simulink model "ctrl_T"  (R2015a)
settings: Solver=ode3  StartTime=0.0  StopTime=inf  FixedStep=0.01  RelTol=1e-3
values from neighbouring files (symbols this model uses):
  C = [C1;C2;C3;C4;C5;C6]    [initfile.m]    (also in thrustallocationQuadraticFixed.m)
  D = 3.0/100    (= 0.03)    [initfile.m]    (also in thrustallocationQuadraticFixed.m = 0.0411111111111)
  eps_c = 5    [initfile.m]
  epsilon = 0.5    [initfile.m]    (also in thrustallocationPseudo.m = u(10); thrustallocationQuadraticFixed.m = u(10))
  hd = c2d(H1,0.01,'foh')    [initfile.m]
  hd2 = c2d(H2,0.01,'zoh')    [initfile.m]
  I_s = 25000 /747225    (= 0.0334571246947)    [initfile.m]
  k_cc = 1    [initfile.m]
  K_omega = 0.3    [initfile.m]
  Kp = 3.3    [initfile.m]
  Max_Acceleration = 5    [initfile.m]
  Max_rotation = 12*sqrt(lambda)    [initfile.m]
  Max_thrust = 1.5    [initfile.m]
  n_c = 5    [initfile.m]
  n_max = 152    [initfile.m]
  p_cc = 0.5    [initfile.m]
  Q_f0 = 0.3    [initfile.m]
  r_cc = 4    [initfile.m]
  Rho = Rho_m    (= 1000)    [initfile.m]
undefined symbols (not defined in the file or in its folder): Kq, Kqr, Kt, Ktr, P_max, Q_max, shaft_to_pwm_coeff, thrust_to_pwm_coeff, Thruster, Thruster_control, Thruster_lock
libraries: simulink x6, marine_gnc x4, simulink_extras x3
(part 3 of 4)

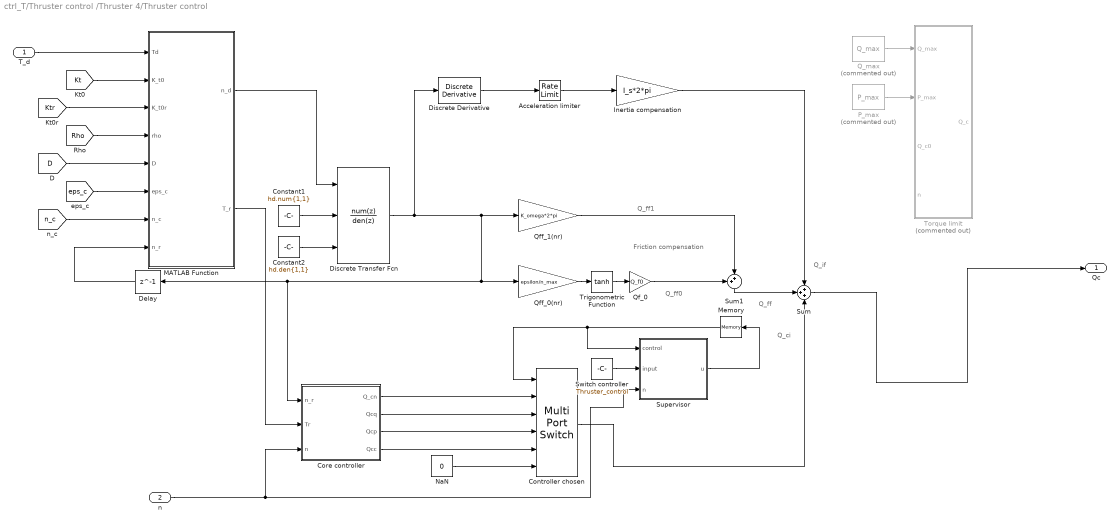
== system ctrl_T/Thruster control /Thruster 4/Thruster control ==
  note: Q_ci
  note: Q_if
  note: Q_ff
  note: Q_ff0
  note: Q_ff1
  note: Friction compensation
  "T_d " : Inport
  n : Inport  Port=2
  Acceleration limiter : RateLimiter  RisingSlewLimit=Max_Acceleration  FallingSlewLimit=-Max_Acceleration  SampleTimeMode=inherited
  Constant1 : Constant  Value=hd.num{1,1}  VectorParams1D=off
  Constant2 : Constant  Value=hd.den{1,1}  VectorParams1D=off
  Controller chosen : MultiPortSwitch  Inputs=5
  Core controller : Subsystem
  Delay : Delay  DelayLength=1  InitialCondition=0
  Discrete Transfer Fcn : DiscreteTransferFcn  NumeratorSource=Input port  Numerator=[8.76e-05 0.0003481 8.648e-05]  DenominatorSource=Input port  Denominator=[1 -1.974 0.9746]  SampleTime=0.01  a0EqualsOne=on
      settings: InputPortMap=u0,p1,p3
  Discrete Derivative : simulink/Discrete/Discrete Derivative  gainval=1.0  ICPrevScaledInput=0.0  InputProcessing=Inherited  OutMin=[]  OutMax=[]  OutDataType=fixdt(1, 16)  OutScaling=2^-10  DoSatur=off
  Inertia compensation : Gain  Gain=I_s*2*pi
  MATLAB Function : MATLAB Function  TreatAsAtomicUnit=on
  Memory : Memory  X0=1
  NaN : Constant  Value=0
  P_max : Constant  Commented=on  Value=P_max
  Q_max : Constant  Commented=on  Value=Q_max
  Qf_0 : Gain  Gain=Q_f0
  Qff_0(nr) : Gain  Gain=epsilon/n_max
  Qff_1(nr) : Gain  Gain=K_omega*2*pi
  Sum : Sum  Inputs=+++
  Sum1 : Sum  Inputs=++|
  Supervisor : MATLAB Function  TreatAsAtomicUnit=on
  Switch controller : Constant  Value=Thruster_control
  Torque limit : MATLAB Function  Commented=on  TreatAsAtomicUnit=on
  Trigonometric Function : Trigonometry  Operator=tanh
  Qc : Outport
  wires:
  P_max/1 -> Torque limit/2(P_max)
  Q_max/1 -> Torque limit/1(Q_max)
  Sum/1 -> Qc/1
  MATLAB Function/2(T_r) -> Core controller/2("Tr ")
  Discrete Derivative/1 -> Acceleration limiter/1
  Qff_0(nr)/1 -> Trigonometric Function/1
  Trigonometric Function/1 -> Qf_0/1
  Sum1/1 -> Sum/2
  Core controller/1(Q_cn) -> Controller chosen/2
  Core controller/4(Qcc) -> Controller chosen/5
  NaN/1 -> Controller chosen/6
  Memory/1 -> Supervisor/1(control), Controller chosen/1
  Qff_1(nr)/1 -> Sum1/2
  Qf_0/1 -> Sum1/1
  Controller chosen/1 -> Sum/3
  Inertia compensation/1 -> Sum/1
  Core controller/3(Qcp) -> Controller chosen/4
  Core controller/2(Qcq) -> Controller chosen/3
  Switch controller/1 -> Supervisor/2(input)
  "T_d "/1 -> MATLAB Function/1(Td)
  [Kt] -> MATLAB Function/2(K_t0)
  [Rho] -> MATLAB Function/4(rho)
  [D] -> MATLAB Function/5(D)
  [eps_c] -> MATLAB Function/6(eps_c)
  [Ktr] -> MATLAB Function/3(K_t0r)
  [n_c] -> MATLAB Function/7(n_c)
  Constant1/1 -> Discrete Transfer Fcn/2
  Constant2/1 -> Discrete Transfer Fcn/3
  MATLAB Function/1(n_d) -> Discrete Transfer Fcn/1
  n/1 -> Supervisor/3(n), Core controller/3("n ")
  Discrete Transfer Fcn/1 -> Discrete Derivative/1, Core controller/1(n_r), Delay/1, Qff_0(nr)/1, Qff_1(nr)/1
  Acceleration limiter/1 -> Inertia compensation/1
  Supervisor/1(u) -> Memory/1
  Delay/1 -> MATLAB Function/8(n_r)

== system ctrl_T/Thruster control /Thruster 5/Propeller Hydrodynamics ==
  env : Inport
  n : Inport  Port=2
  Actual Force and Torque : MATLAB Function  TreatAsAtomicUnit=on
  Ta : Outport
  Qa : Outport  Port=2
  wires:
  n/1 -> Actual Force and Torque/1(n)
  [D] -> Actual Force and Torque/7(D)
  [Kq] -> Actual Force and Torque/2(Kq)
  Actual Force and Torque/2(Qa) -> Qa/1
  [Rho] -> Actual Force and Torque/6(Rho)
  env/1 -> Actual Force and Torque/9(env)
  [Kt] -> Actual Force and Torque/3(Kt)
  Actual Force and Torque/1(Ta) -> Ta/1
  [Ktr] -> Actual Force and Torque/4(Ktr)
  [Kqr] -> Actual Force and Torque/5(Kqr)
  [eps_c] -> Actual Force and Torque/8(eps_c)

== system ctrl_T/Thruster control /Thruster 5/Shaft dynamics ==
  Qm : Inport
  Qa : Inport  Port=2
  Finding rotation speed : Gain  Gain=1/(2*pi*I_s)
  Integrator : Integrator  ExternalReset=either
  K_omega : Gain  Gain=K_omega*2*pi
  Sum : Sum  Inputs=-+-
  reset : S-Function  Priority=1  FunctionName=NIVeriStandIO  Parameters=width dtype portnum stime stype btype  mask(NI VeriStand Inport){portnum=1, width=-1, stime=-1, dtype=auto, stype=auto, btype=1}
      mask prompts: portnum "Port number:"; width "Port dimensions (-1 for dynamically sized):"; stime "Sample time (-1 for inherited):"; dtype "Data type:"; stype "Signal type:"; btype "Block type:"
      mask help: Use this inport on any level of nested subsystems to allow NI VeriStand software to map signals to it.
      mask init:
      | NIVeriStandIO_init;
      settings: CopyFcn=NIVeriStand_MDL_functions('', 'IO_copy');  DeleteFcn=NIVeriStand_MDL_functions('', 'IO_delete');  MoveFcn=set_param(gcb, 'Mask', 'on');
      mask Callback portnum: NIVeriStand_MDL_functions('', 'IO_setportnum');
      mask TypeOptions dtype: auto | double | single | int8 | uint8 | int16 | uint16 | int32 | uint32 | boolean
      mask Callback dtype: NIVeriStand_MDL_functions('', 'IO_booleansignal');
      mask TypeOptions stype: auto | real | complex
      mask Display:
      | patch([-x x], [-y y], [.90980 .81960 .32156]);
      | plot([xrad -x x xrad], [yrad -y y yrad]);
      | fprintf('NI In%d', portnum);
  n : Outport
  wires:
  Qm/1 -> Sum/2
  Sum/1 -> Finding rotation speed/1
  Qa/1 -> Sum/1
  K_omega/1 -> Sum/3
  Finding rotation speed/1 -> Integrator/1
  Integrator/1 -> K_omega/1, n/1
  reset/1 -> Integrator/2

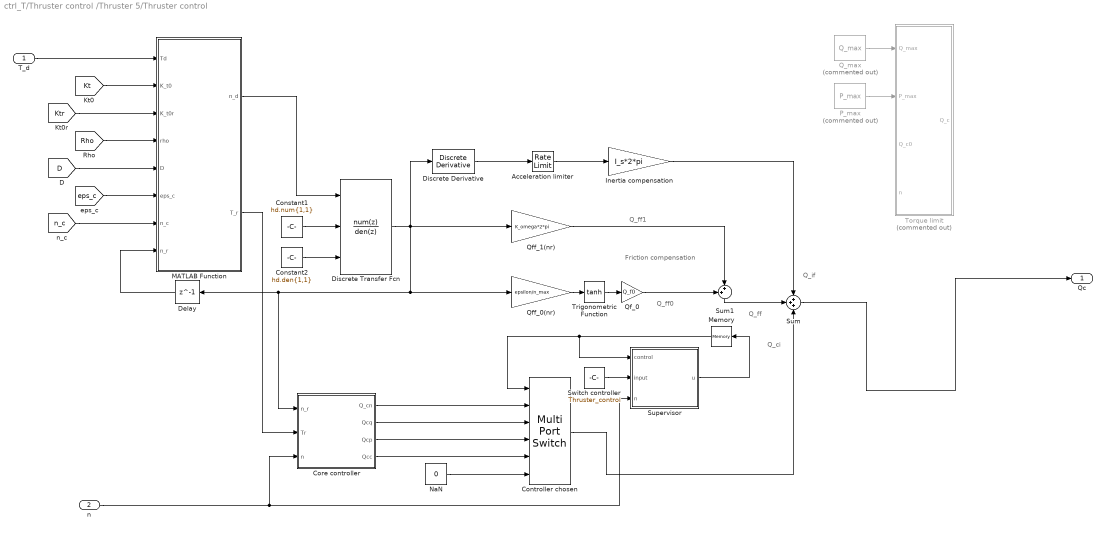
== system ctrl_T/Thruster control /Thruster 5/Thruster control ==
  note: Q_ci
  note: Q_if
  note: Q_ff
  note: Q_ff0
  note: Q_ff1
  note: Friction compensation
  "T_d " : Inport
  n : Inport  Port=2
  Acceleration limiter : RateLimiter  RisingSlewLimit=Max_Acceleration  FallingSlewLimit=-Max_Acceleration  SampleTimeMode=inherited
  Constant1 : Constant  Value=hd.num{1,1}  VectorParams1D=off
  Constant2 : Constant  Value=hd.den{1,1}  VectorParams1D=off
  Controller chosen : MultiPortSwitch  Inputs=5
  Core controller : Subsystem
  Delay : Delay  DelayLength=1  InitialCondition=0
  Discrete Transfer Fcn : DiscreteTransferFcn  NumeratorSource=Input port  Numerator=[8.76e-05 0.0003481 8.648e-05]  DenominatorSource=Input port  Denominator=[1 -1.974 0.9746]  SampleTime=0.01  a0EqualsOne=on
      settings: InputPortMap=u0,p1,p3
  Discrete Derivative : simulink/Discrete/Discrete Derivative  gainval=1.0  ICPrevScaledInput=0.0  InputProcessing=Inherited  OutMin=[]  OutMax=[]  OutDataType=fixdt(1, 16)  OutScaling=2^-10  DoSatur=off
  Inertia compensation : Gain  Gain=I_s*2*pi
  MATLAB Function : MATLAB Function  TreatAsAtomicUnit=on
  Memory : Memory  X0=1
  NaN : Constant  Value=0
  P_max : Constant  Commented=on  Value=P_max
  Q_max : Constant  Commented=on  Value=Q_max
  Qf_0 : Gain  Gain=Q_f0
  Qff_0(nr) : Gain  Gain=epsilon/n_max
  Qff_1(nr) : Gain  Gain=K_omega*2*pi
  Sum : Sum  Inputs=+++
  Sum1 : Sum  Inputs=++|
  Supervisor : MATLAB Function  TreatAsAtomicUnit=on
  Switch controller : Constant  Value=Thruster_control
  Torque limit : MATLAB Function  Commented=on  TreatAsAtomicUnit=on
  Trigonometric Function : Trigonometry  Operator=tanh
  Qc : Outport
  wires:
  P_max/1 -> Torque limit/2(P_max)
  Q_max/1 -> Torque limit/1(Q_max)
  Sum/1 -> Qc/1
  MATLAB Function/2(T_r) -> Core controller/2("Tr ")
  Discrete Derivative/1 -> Acceleration limiter/1
  Qff_0(nr)/1 -> Trigonometric Function/1
  Trigonometric Function/1 -> Qf_0/1
  Sum1/1 -> Sum/2
  Core controller/1(Q_cn) -> Controller chosen/2
  Core controller/4(Qcc) -> Controller chosen/5
  NaN/1 -> Controller chosen/6
  Memory/1 -> Supervisor/1(control), Controller chosen/1
  Qff_1(nr)/1 -> Sum1/2
  Qf_0/1 -> Sum1/1
  Controller chosen/1 -> Sum/3
  Inertia compensation/1 -> Sum/1
  Core controller/3(Qcp) -> Controller chosen/4
  Core controller/2(Qcq) -> Controller chosen/3
  Switch controller/1 -> Supervisor/2(input)
  "T_d "/1 -> MATLAB Function/1(Td)
  [Kt] -> MATLAB Function/2(K_t0)
  [Rho] -> MATLAB Function/4(rho)
  [D] -> MATLAB Function/5(D)
  [eps_c] -> MATLAB Function/6(eps_c)
  [Ktr] -> MATLAB Function/3(K_t0r)
  [n_c] -> MATLAB Function/7(n_c)
  Constant1/1 -> Discrete Transfer Fcn/2
  Constant2/1 -> Discrete Transfer Fcn/3
  MATLAB Function/1(n_d) -> Discrete Transfer Fcn/1
  Discrete Transfer Fcn/1 -> Discrete Derivative/1, Qff_0(nr)/1, Core controller/1(n_r), Delay/1, Qff_1(nr)/1
  Acceleration limiter/1 -> Inertia compensation/1
  Supervisor/1(u) -> Memory/1
  Delay/1 -> MATLAB Function/8(n_r)
  n/1 -> Core controller/3("n "), Supervisor/3(n)

== system ctrl_T/Thruster control /Thruster 6/Propeller Hydrodynamics ==
  env : Inport
  n : Inport  Port=2
  Actual Force and Torque : MATLAB Function  TreatAsAtomicUnit=on
  Ta : Outport
  Qa : Outport  Port=2
  wires:
  n/1 -> Actual Force and Torque/1(n)
  [D] -> Actual Force and Torque/7(D)
  [Kq] -> Actual Force and Torque/2(Kq)
  Actual Force and Torque/2(Qa) -> Qa/1
  [Rho] -> Actual Force and Torque/6(Rho)
  env/1 -> Actual Force and Torque/9(env)
  [Kt] -> Actual Force and Torque/3(Kt)
  Actual Force and Torque/1(Ta) -> Ta/1
  [Ktr] -> Actual Force and Torque/4(Ktr)
  [Kqr] -> Actual Force and Torque/5(Kqr)
  [eps_c] -> Actual Force and Torque/8(eps_c)

== system ctrl_T/Thruster control /Thruster 6/Shaft dynamics ==
  Qm : Inport
  Qa : Inport  Port=2
  Finding rotation speed : Gain  Gain=1/(2*pi*I_s)
  Integrator : Integrator  ExternalReset=either
  K_omega : Gain  Gain=K_omega*2*pi
  Sum : Sum  Inputs=-+-
  reset : S-Function  Priority=1  FunctionName=NIVeriStandIO  Parameters=width dtype portnum stime stype btype  mask(NI VeriStand Inport){portnum=1, width=-1, stime=-1, dtype=auto, stype=auto, btype=1}
      mask prompts: portnum "Port number:"; width "Port dimensions (-1 for dynamically sized):"; stime "Sample time (-1 for inherited):"; dtype "Data type:"; stype "Signal type:"; btype "Block type:"
      mask help: Use this inport on any level of nested subsystems to allow NI VeriStand software to map signals to it.
      mask init:
      | NIVeriStandIO_init;
      settings: CopyFcn=NIVeriStand_MDL_functions('', 'IO_copy');  DeleteFcn=NIVeriStand_MDL_functions('', 'IO_delete');  MoveFcn=set_param(gcb, 'Mask', 'on');
      mask Callback portnum: NIVeriStand_MDL_functions('', 'IO_setportnum');
      mask TypeOptions dtype: auto | double | single | int8 | uint8 | int16 | uint16 | int32 | uint32 | boolean
      mask Callback dtype: NIVeriStand_MDL_functions('', 'IO_booleansignal');
      mask TypeOptions stype: auto | real | complex
      mask Display:
      | patch([-x x], [-y y], [.90980 .81960 .32156]);
      | plot([xrad -x x xrad], [yrad -y y yrad]);
      | fprintf('NI In%d', portnum);
  n : Outport
  wires:
  Qm/1 -> Sum/2
  Sum/1 -> Finding rotation speed/1
  Qa/1 -> Sum/1
  K_omega/1 -> Sum/3
  Integrator/1 -> K_omega/1, n/1
  reset/1 -> Integrator/2
  Finding rotation speed/1 -> Integrator/1

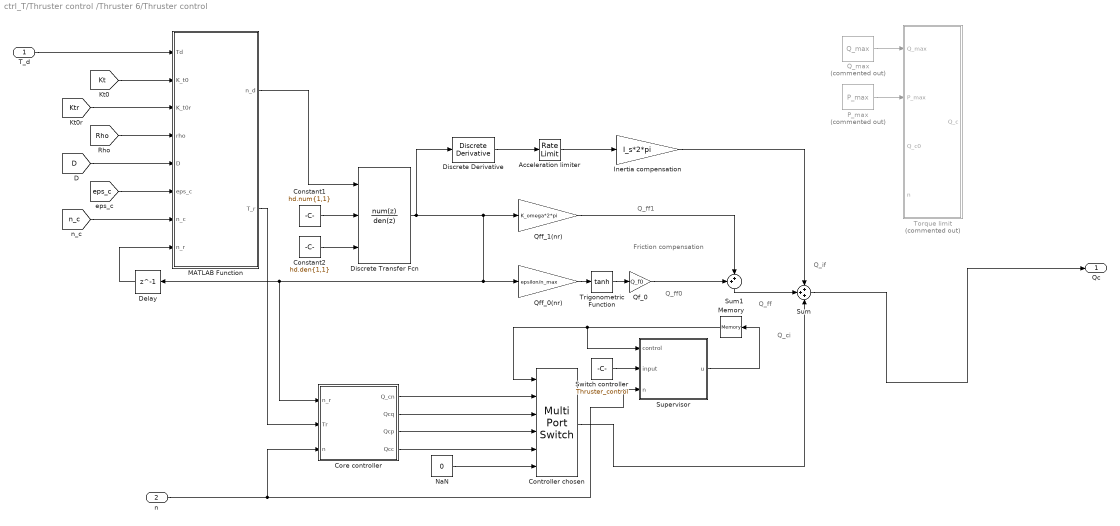
== system ctrl_T/Thruster control /Thruster 6/Thruster control ==
  note: Q_ci
  note: Q_if
  note: Q_ff
  note: Q_ff0
  note: Q_ff1
  note: Friction compensation
  "T_d " : Inport
  n : Inport  Port=2
  Acceleration limiter : RateLimiter  RisingSlewLimit=Max_Acceleration  FallingSlewLimit=-Max_Acceleration  SampleTimeMode=inherited
  Constant1 : Constant  Value=hd.num{1,1}  VectorParams1D=off
  Constant2 : Constant  Value=hd.den{1,1}  VectorParams1D=off
  Controller chosen : MultiPortSwitch  Inputs=5
  Core controller : Subsystem
  Delay : Delay  DelayLength=1  InitialCondition=0
  Discrete Transfer Fcn : DiscreteTransferFcn  NumeratorSource=Input port  Numerator=[8.76e-05 0.0003481 8.648e-05]  DenominatorSource=Input port  Denominator=[1 -1.974 0.9746]  SampleTime=0.01  a0EqualsOne=on
      settings: InputPortMap=u0,p1,p3
  Discrete Derivative : simulink/Discrete/Discrete Derivative  gainval=1.0  ICPrevScaledInput=0.0  InputProcessing=Inherited  OutMin=[]  OutMax=[]  OutDataType=fixdt(1, 16)  OutScaling=2^-10  DoSatur=off
  Inertia compensation : Gain  Gain=I_s*2*pi
  MATLAB Function : MATLAB Function  TreatAsAtomicUnit=on
  Memory : Memory  X0=1
  NaN : Constant  Value=0
  P_max : Constant  Commented=on  Value=P_max
  Q_max : Constant  Commented=on  Value=Q_max
  Qf_0 : Gain  Gain=Q_f0
  Qff_0(nr) : Gain  Gain=epsilon/n_max
  Qff_1(nr) : Gain  Gain=K_omega*2*pi
  Sum : Sum  Inputs=+++
  Sum1 : Sum  Inputs=++|
  Supervisor : MATLAB Function  TreatAsAtomicUnit=on
  Switch controller : Constant  Value=Thruster_control
  Torque limit : MATLAB Function  Commented=on  TreatAsAtomicUnit=on
  Trigonometric Function : Trigonometry  Operator=tanh
  Qc : Outport
  wires:
  P_max/1 -> Torque limit/2(P_max)
  Q_max/1 -> Torque limit/1(Q_max)
  Sum/1 -> Qc/1
  MATLAB Function/2(T_r) -> Core controller/2("Tr ")
  Discrete Derivative/1 -> Acceleration limiter/1
  Qff_0(nr)/1 -> Trigonometric Function/1
  Trigonometric Function/1 -> Qf_0/1
  Sum1/1 -> Sum/2
  Core controller/1(Q_cn) -> Controller chosen/2
  Core controller/4(Qcc) -> Controller chosen/5
  NaN/1 -> Controller chosen/6
  Memory/1 -> Supervisor/1(control), Controller chosen/1
  Qff_1(nr)/1 -> Sum1/2
  Qf_0/1 -> Sum1/1
  Controller chosen/1 -> Sum/3
  Inertia compensation/1 -> Sum/1
  Core controller/3(Qcp) -> Controller chosen/4
  Core controller/2(Qcq) -> Controller chosen/3
  Switch controller/1 -> Supervisor/2(input)
  "T_d "/1 -> MATLAB Function/1(Td)
  [Kt] -> MATLAB Function/2(K_t0)
  [Rho] -> MATLAB Function/4(rho)
  [D] -> MATLAB Function/5(D)
  [eps_c] -> MATLAB Function/6(eps_c)
  [Ktr] -> MATLAB Function/3(K_t0r)
  [n_c] -> MATLAB Function/7(n_c)
  Constant1/1 -> Discrete Transfer Fcn/2
  Constant2/1 -> Discrete Transfer Fcn/3
  MATLAB Function/1(n_d) -> Discrete Transfer Fcn/1
  n/1 -> Supervisor/3(n), Core controller/3("n ")
  Discrete Transfer Fcn/1 -> Discrete Derivative/1, Core controller/1(n_r), Delay/1, Qff_0(nr)/1, Qff_1(nr)/1
  Acceleration limiter/1 -> Inertia compensation/1
  Supervisor/1(u) -> Memory/1
  Delay/1 -> MATLAB Function/8(n_r)

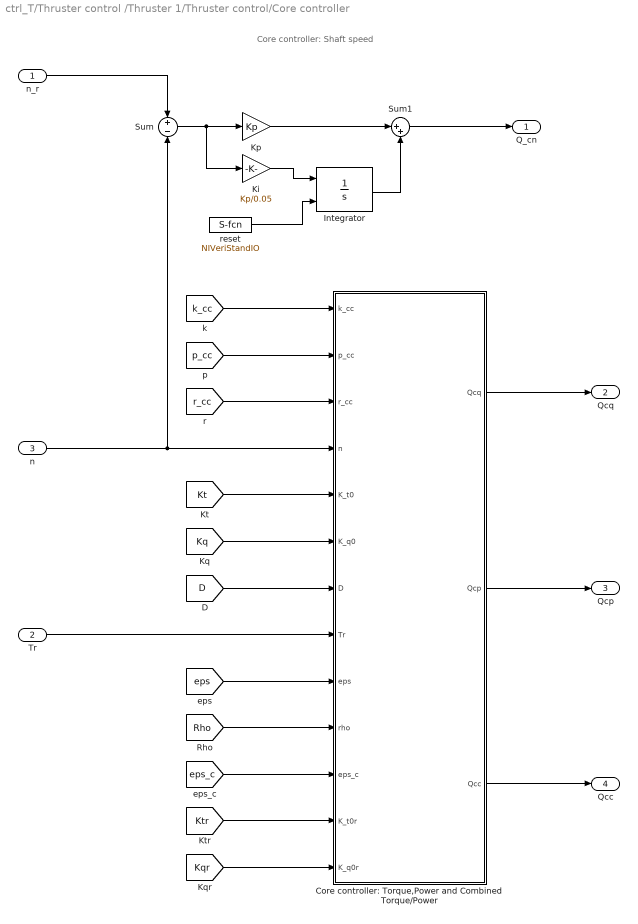
== system ctrl_T/Thruster control /Thruster 1/Thruster control/Core controller ==
  note: Core controller: Shaft speed
  n_r : Inport
  "Tr " : Inport  Port=2
  "n " : Inport  Port=3
  Core controller: Torque,Power and Combined Torque/Power : MATLAB Function  TreatAsAtomicUnit=on
  Integrator : Integrator  ExternalReset=either  UpperSaturationLimit=Q_max  LowerSaturationLimit=-Q_max
  Ki : Gain  Gain=Kp/0.05
  Kp : Gain  Gain=Kp
  Sum : Sum  Inputs=+|-
  Sum1 : Sum  Inputs=|++
  reset : S-Function  Priority=1  FunctionName=NIVeriStandIO  Parameters=width dtype portnum stime stype btype  mask(NI VeriStand Inport){portnum=1, width=-1, stime=-1, dtype=auto, stype=auto, btype=1}
      mask prompts: portnum "Port number:"; width "Port dimensions (-1 for dynamically sized):"; stime "Sample time (-1 for inherited):"; dtype "Data type:"; stype "Signal type:"; btype "Block type:"
      mask help: Use this inport on any level of nested subsystems to allow NI VeriStand software to map signals to it.
      mask init:
      | NIVeriStandIO_init;
      settings: CopyFcn=NIVeriStand_MDL_functions('', 'IO_copy');  DeleteFcn=NIVeriStand_MDL_functions('', 'IO_delete');  MoveFcn=set_param(gcb, 'Mask', 'on');
      mask Callback portnum: NIVeriStand_MDL_functions('', 'IO_setportnum');
      mask TypeOptions dtype: auto | double | single | int8 | uint8 | int16 | uint16 | int32 | uint32 | boolean
      mask Callback dtype: NIVeriStand_MDL_functions('', 'IO_booleansignal');
      mask TypeOptions stype: auto | real | complex
      mask Display:
      | patch([-x x], [-y y], [.90980 .81960 .32156]);
      | plot([xrad -x x xrad], [yrad -y y yrad]);
      | fprintf('NI In%d', portnum);
  Q_cn : Outport
  Qcq : Outport  Port=2
  Qcp : Outport  Port=3
  Qcc : Outport  Port=4
  wires:
  [k_cc] -> Core controller: Torque,Power and Combined Torque/Power/1(k_cc)
  [p_cc] -> Core controller: Torque,Power and Combined Torque/Power/2(p_cc)
  [r_cc] -> Core controller: Torque,Power and Combined Torque/Power/3(r_cc)
  Core controller: Torque,Power and Combined Torque/Power/3(Qcc) -> Qcc/1
  [Kt] -> Core controller: Torque,Power and Combined Torque/Power/5(K_t0)
  [D] -> Core controller: Torque,Power and Combined Torque/Power/7(D)
  [Kq] -> Core controller: Torque,Power and Combined Torque/Power/6(K_q0)
  [Rho] -> Core controller: Torque,Power and Combined Torque/Power/10(rho)
  [eps] -> Core controller: Torque,Power and Combined Torque/Power/9(eps)
  "n "/1 -> Sum/2, Core controller: Torque,Power and Combined Torque/Power/4(n)
  "Tr "/1 -> Core controller: Torque,Power and Combined Torque/Power/8(Tr)
  Core controller: Torque,Power and Combined Torque/Power/2(Qcp) -> Qcp/1
  Core controller: Torque,Power and Combined Torque/Power/1(Qcq) -> Qcq/1
  n_r/1 -> Sum/1
  Ki/1 -> Integrator/1
  Kp/1 -> Sum1/1
  Integrator/1 -> Sum1/2
  Sum1/1 -> Q_cn/1
  Sum/1 -> Ki/1, Kp/1
  reset/1 -> Integrator/2
  [eps_c] -> Core controller: Torque,Power and Combined Torque/Power/11(eps_c)
  [Ktr] -> Core controller: Torque,Power and Combined Torque/Power/12(K_t0r)
  [Kqr] -> Core controller: Torque,Power and Combined Torque/Power/13(K_q0r)

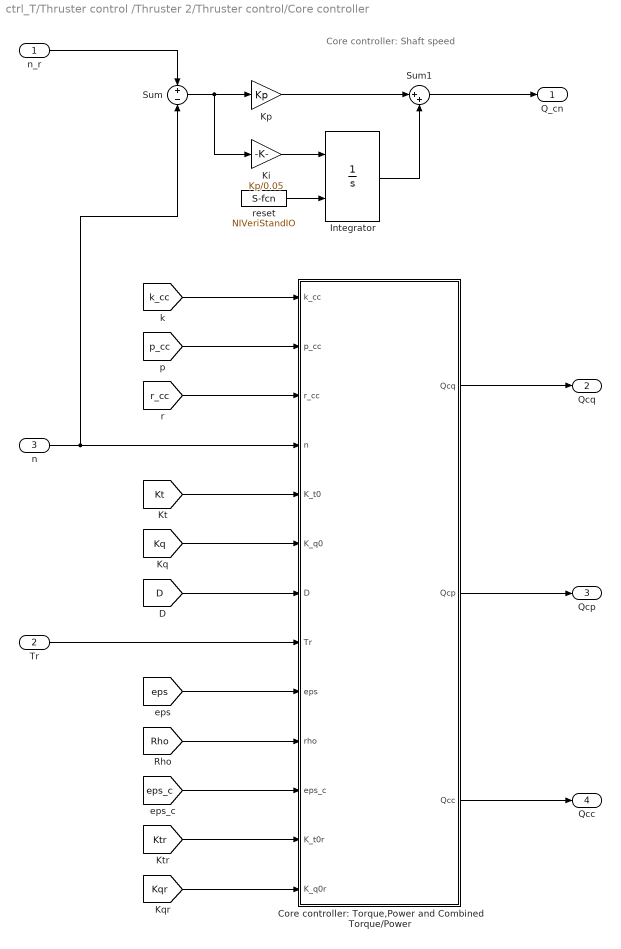
== system ctrl_T/Thruster control /Thruster 2/Thruster control/Core controller ==
  note: Core controller: Shaft speed
  n_r : Inport
  "Tr " : Inport  Port=2
  "n " : Inport  Port=3
  Core controller: Torque,Power and Combined Torque/Power : MATLAB Function  TreatAsAtomicUnit=on
  Integrator : Integrator  ExternalReset=either  UpperSaturationLimit=Q_max  LowerSaturationLimit=-Q_max
  Ki : Gain  Gain=Kp/0.05
  Kp : Gain  Gain=Kp
  Sum : Sum  Inputs=+|-
  Sum1 : Sum  Inputs=|++
  reset : S-Function  Priority=1  FunctionName=NIVeriStandIO  Parameters=width dtype portnum stime stype btype  mask(NI VeriStand Inport){portnum=1, width=-1, stime=-1, dtype=auto, stype=auto, btype=1}
      mask prompts: portnum "Port number:"; width "Port dimensions (-1 for dynamically sized):"; stime "Sample time (-1 for inherited):"; dtype "Data type:"; stype "Signal type:"; btype "Block type:"
      mask help: Use this inport on any level of nested subsystems to allow NI VeriStand software to map signals to it.
      mask init:
      | NIVeriStandIO_init;
      settings: CopyFcn=NIVeriStand_MDL_functions('', 'IO_copy');  DeleteFcn=NIVeriStand_MDL_functions('', 'IO_delete');  MoveFcn=set_param(gcb, 'Mask', 'on');
      mask Callback portnum: NIVeriStand_MDL_functions('', 'IO_setportnum');
      mask TypeOptions dtype: auto | double | single | int8 | uint8 | int16 | uint16 | int32 | uint32 | boolean
      mask Callback dtype: NIVeriStand_MDL_functions('', 'IO_booleansignal');
      mask TypeOptions stype: auto | real | complex
      mask Display:
      | patch([-x x], [-y y], [.90980 .81960 .32156]);
      | plot([xrad -x x xrad], [yrad -y y yrad]);
      | fprintf('NI In%d', portnum);
  Q_cn : Outport
  Qcq : Outport  Port=2
  Qcp : Outport  Port=3
  Qcc : Outport  Port=4
  wires:
  n_r/1 -> Sum/1
  Ki/1 -> Integrator/1
  Kp/1 -> Sum1/1
  Integrator/1 -> Sum1/2
  Sum/1 -> Ki/1, Kp/1
  Sum1/1 -> Q_cn/1
  reset/1 -> Integrator/2
  [k_cc] -> Core controller: Torque,Power and Combined Torque/Power/1(k_cc)
  [p_cc] -> Core controller: Torque,Power and Combined Torque/Power/2(p_cc)
  [r_cc] -> Core controller: Torque,Power and Combined Torque/Power/3(r_cc)
  Core controller: Torque,Power and Combined Torque/Power/3(Qcc) -> Qcc/1
  [Kt] -> Core controller: Torque,Power and Combined Torque/Power/5(K_t0)
  [D] -> Core controller: Torque,Power and Combined Torque/Power/7(D)
  [Kq] -> Core controller: Torque,Power and Combined Torque/Power/6(K_q0)
  [Rho] -> Core controller: Torque,Power and Combined Torque/Power/10(rho)
  [eps] -> Core controller: Torque,Power and Combined Torque/Power/9(eps)
  "n "/1 -> Core controller: Torque,Power and Combined Torque/Power/4(n), Sum/2
  "Tr "/1 -> Core controller: Torque,Power and Combined Torque/Power/8(Tr)
  Core controller: Torque,Power and Combined Torque/Power/2(Qcp) -> Qcp/1
  Core controller: Torque,Power and Combined Torque/Power/1(Qcq) -> Qcq/1
  [eps_c] -> Core controller: Torque,Power and Combined Torque/Power/11(eps_c)
  [Ktr] -> Core controller: Torque,Power and Combined Torque/Power/12(K_t0r)
  [Kqr] -> Core controller: Torque,Power and Combined Torque/Power/13(K_q0r)

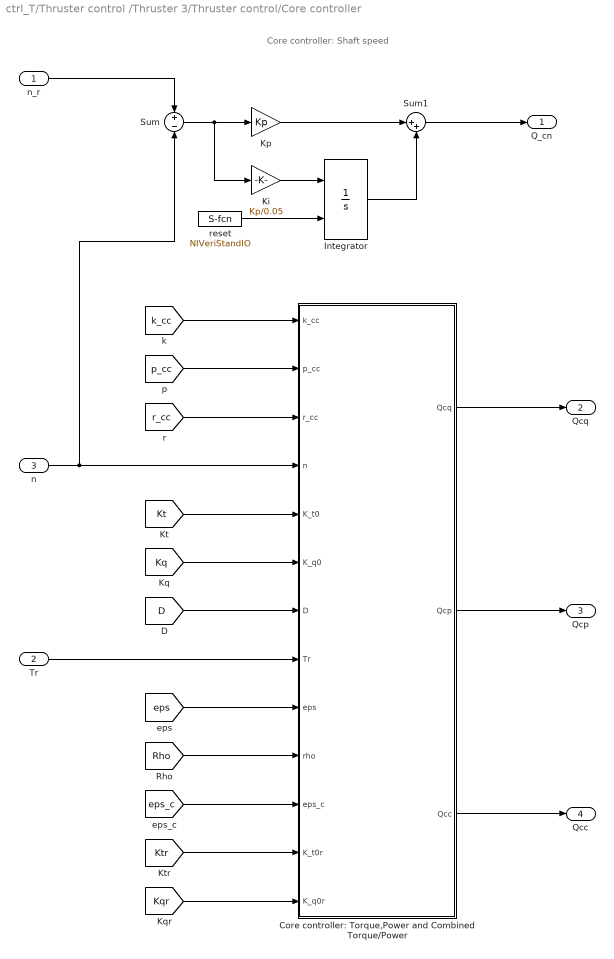
== system ctrl_T/Thruster control /Thruster 3/Thruster control/Core controller ==
  note: Core controller: Shaft speed
  n_r : Inport
  "Tr " : Inport  Port=2
  "n " : Inport  Port=3
  Core controller: Torque,Power and Combined Torque/Power : MATLAB Function  TreatAsAtomicUnit=on
  Integrator : Integrator  ExternalReset=either  UpperSaturationLimit=Q_max  LowerSaturationLimit=-Q_max
  Ki : Gain  Gain=Kp/0.05
  Kp : Gain  Gain=Kp
  Sum : Sum  Inputs=+|-
  Sum1 : Sum  Inputs=|++
  reset : S-Function  Priority=1  FunctionName=NIVeriStandIO  Parameters=width dtype portnum stime stype btype  mask(NI VeriStand Inport){portnum=1, width=-1, stime=-1, dtype=auto, stype=auto, btype=1}
      mask prompts: portnum "Port number:"; width "Port dimensions (-1 for dynamically sized):"; stime "Sample time (-1 for inherited):"; dtype "Data type:"; stype "Signal type:"; btype "Block type:"
      mask help: Use this inport on any level of nested subsystems to allow NI VeriStand software to map signals to it.
      mask init:
      | NIVeriStandIO_init;
      settings: CopyFcn=NIVeriStand_MDL_functions('', 'IO_copy');  DeleteFcn=NIVeriStand_MDL_functions('', 'IO_delete');  MoveFcn=set_param(gcb, 'Mask', 'on');
      mask Callback portnum: NIVeriStand_MDL_functions('', 'IO_setportnum');
      mask TypeOptions dtype: auto | double | single | int8 | uint8 | int16 | uint16 | int32 | uint32 | boolean
      mask Callback dtype: NIVeriStand_MDL_functions('', 'IO_booleansignal');
      mask TypeOptions stype: auto | real | complex
      mask Display:
      | patch([-x x], [-y y], [.90980 .81960 .32156]);
      | plot([xrad -x x xrad], [yrad -y y yrad]);
      | fprintf('NI In%d', portnum);
  Q_cn : Outport
  Qcq : Outport  Port=2
  Qcp : Outport  Port=3
  Qcc : Outport  Port=4
  wires:
  n_r/1 -> Sum/1
  Ki/1 -> Integrator/1
  Kp/1 -> Sum1/1
  Integrator/1 -> Sum1/2
  Sum/1 -> Ki/1, Kp/1
  Sum1/1 -> Q_cn/1
  reset/1 -> Integrator/2
  [k_cc] -> Core controller: Torque,Power and Combined Torque/Power/1(k_cc)
  [p_cc] -> Core controller: Torque,Power and Combined Torque/Power/2(p_cc)
  [r_cc] -> Core controller: Torque,Power and Combined Torque/Power/3(r_cc)
  Core controller: Torque,Power and Combined Torque/Power/3(Qcc) -> Qcc/1
  [Kt] -> Core controller: Torque,Power and Combined Torque/Power/5(K_t0)
  [D] -> Core controller: Torque,Power and Combined Torque/Power/7(D)
  [Kq] -> Core controller: Torque,Power and Combined Torque/Power/6(K_q0)
  [Rho] -> Core controller: Torque,Power and Combined Torque/Power/10(rho)
  [eps] -> Core controller: Torque,Power and Combined Torque/Power/9(eps)
  "n "/1 -> Sum/2, Core controller: Torque,Power and Combined Torque/Power/4(n)
  "Tr "/1 -> Core controller: Torque,Power and Combined Torque/Power/8(Tr)
  Core controller: Torque,Power and Combined Torque/Power/2(Qcp) -> Qcp/1
  Core controller: Torque,Power and Combined Torque/Power/1(Qcq) -> Qcq/1
  [eps_c] -> Core controller: Torque,Power and Combined Torque/Power/11(eps_c)
  [Ktr] -> Core controller: Torque,Power and Combined Torque/Power/12(K_t0r)
  [Kqr] -> Core controller: Torque,Power and Combined Torque/Power/13(K_q0r)

== system ctrl_T/Thruster control /Thruster 4/Thruster control/Core controller ==
  note: Core controller: Shaft speed
  n_r : Inport
  "Tr " : Inport  Port=2
  "n " : Inport  Port=3
  Core controller: Torque,Power and Combined Torque/Power : MATLAB Function  TreatAsAtomicUnit=on
  Integrator : Integrator  ExternalReset=either  UpperSaturationLimit=Q_max  LowerSaturationLimit=-Q_max
  Ki : Gain  Gain=Kp/0.05
  Kp : Gain  Gain=Kp
  Sum : Sum  Inputs=+|-
  Sum1 : Sum  Inputs=|++
  reset : S-Function  Priority=1  FunctionName=NIVeriStandIO  Parameters=width dtype portnum stime stype btype  mask(NI VeriStand Inport){portnum=1, width=-1, stime=-1, dtype=auto, stype=auto, btype=1}
      mask prompts: portnum "Port number:"; width "Port dimensions (-1 for dynamically sized):"; stime "Sample time (-1 for inherited):"; dtype "Data type:"; stype "Signal type:"; btype "Block type:"
      mask help: Use this inport on any level of nested subsystems to allow NI VeriStand software to map signals to it.
      mask init:
      | NIVeriStandIO_init;
      settings: CopyFcn=NIVeriStand_MDL_functions('', 'IO_copy');  DeleteFcn=NIVeriStand_MDL_functions('', 'IO_delete');  MoveFcn=set_param(gcb, 'Mask', 'on');
      mask Callback portnum: NIVeriStand_MDL_functions('', 'IO_setportnum');
      mask TypeOptions dtype: auto | double | single | int8 | uint8 | int16 | uint16 | int32 | uint32 | boolean
      mask Callback dtype: NIVeriStand_MDL_functions('', 'IO_booleansignal');
      mask TypeOptions stype: auto | real | complex
      mask Display:
      | patch([-x x], [-y y], [.90980 .81960 .32156]);
      | plot([xrad -x x xrad], [yrad -y y yrad]);
      | fprintf('NI In%d', portnum);
  Q_cn : Outport
  Qcq : Outport  Port=2
  Qcp : Outport  Port=3
  Qcc : Outport  Port=4
  wires:
  n_r/1 -> Sum/1
  Ki/1 -> Integrator/1
  Kp/1 -> Sum1/1
  Integrator/1 -> Sum1/2
  Sum/1 -> Ki/1, Kp/1
  Sum1/1 -> Q_cn/1
  [k_cc] -> Core controller: Torque,Power and Combined Torque/Power/1(k_cc)
  [p_cc] -> Core controller: Torque,Power and Combined Torque/Power/2(p_cc)
  [r_cc] -> Core controller: Torque,Power and Combined Torque/Power/3(r_cc)
  Core controller: Torque,Power and Combined Torque/Power/3(Qcc) -> Qcc/1
  [Kt] -> Core controller: Torque,Power and Combined Torque/Power/5(K_t0)
  [D] -> Core controller: Torque,Power and Combined Torque/Power/7(D)
  [Kq] -> Core controller: Torque,Power and Combined Torque/Power/6(K_q0)
  [Rho] -> Core controller: Torque,Power and Combined Torque/Power/10(rho)
  [eps] -> Core controller: Torque,Power and Combined Torque/Power/9(eps)
  "n "/1 -> Core controller: Torque,Power and Combined Torque/Power/4(n), Sum/2
  "Tr "/1 -> Core controller: Torque,Power and Combined Torque/Power/8(Tr)
  Core controller: Torque,Power and Combined Torque/Power/2(Qcp) -> Qcp/1
  Core controller: Torque,Power and Combined Torque/Power/1(Qcq) -> Qcq/1
  [eps_c] -> Core controller: Torque,Power and Combined Torque/Power/11(eps_c)
  [Ktr] -> Core controller: Torque,Power and Combined Torque/Power/12(K_t0r)
  [Kqr] -> Core controller: Torque,Power and Combined Torque/Power/13(K_q0r)
  reset/1 -> Integrator/2

== system ctrl_T/Thruster control /Thruster 5/Thruster control/Core controller ==
  note: Core controller: Shaft speed
  n_r : Inport
  "Tr " : Inport  Port=2
  "n " : Inport  Port=3
  Core controller: Torque,Power and Combined Torque/Power : MATLAB Function  TreatAsAtomicUnit=on
  Integrator : Integrator  ExternalReset=either  UpperSaturationLimit=Q_max  LowerSaturationLimit=-Q_max
  Ki : Gain  Gain=Kp/0.05
  Kp : Gain  Gain=Kp
  Sum : Sum  Inputs=+|-
  Sum1 : Sum  Inputs=|++
  reset : S-Function  Priority=1  FunctionName=NIVeriStandIO  Parameters=width dtype portnum stime stype btype  mask(NI VeriStand Inport){portnum=1, width=-1, stime=-1, dtype=auto, stype=auto, btype=1}
      mask prompts: portnum "Port number:"; width "Port dimensions (-1 for dynamically sized):"; stime "Sample time (-1 for inherited):"; dtype "Data type:"; stype "Signal type:"; btype "Block type:"
      mask help: Use this inport on any level of nested subsystems to allow NI VeriStand software to map signals to it.
      mask init:
      | NIVeriStandIO_init;
      settings: CopyFcn=NIVeriStand_MDL_functions('', 'IO_copy');  DeleteFcn=NIVeriStand_MDL_functions('', 'IO_delete');  MoveFcn=set_param(gcb, 'Mask', 'on');
      mask Callback portnum: NIVeriStand_MDL_functions('', 'IO_setportnum');
      mask TypeOptions dtype: auto | double | single | int8 | uint8 | int16 | uint16 | int32 | uint32 | boolean
      mask Callback dtype: NIVeriStand_MDL_functions('', 'IO_booleansignal');
      mask TypeOptions stype: auto | real | complex
      mask Display:
      | patch([-x x], [-y y], [.90980 .81960 .32156]);
      | plot([xrad -x x xrad], [yrad -y y yrad]);
      | fprintf('NI In%d', portnum);
  Q_cn : Outport
  Qcq : Outport  Port=2
  Qcp : Outport  Port=3
  Qcc : Outport  Port=4
  wires:
  n_r/1 -> Sum/1
  Ki/1 -> Integrator/1
  Kp/1 -> Sum1/1
  Integrator/1 -> Sum1/2
  Sum/1 -> Ki/1, Kp/1
  Sum1/1 -> Q_cn/1
  reset/1 -> Integrator/2
  [k_cc] -> Core controller: Torque,Power and Combined Torque/Power/1(k_cc)
  [p_cc] -> Core controller: Torque,Power and Combined Torque/Power/2(p_cc)
  [r_cc] -> Core controller: Torque,Power and Combined Torque/Power/3(r_cc)
  Core controller: Torque,Power and Combined Torque/Power/3(Qcc) -> Qcc/1
  [Kt] -> Core controller: Torque,Power and Combined Torque/Power/5(K_t0)
  [D] -> Core controller: Torque,Power and Combined Torque/Power/7(D)
  [Kq] -> Core controller: Torque,Power and Combined Torque/Power/6(K_q0)
  [Rho] -> Core controller: Torque,Power and Combined Torque/Power/10(rho)
  [eps] -> Core controller: Torque,Power and Combined Torque/Power/9(eps)
  "n "/1 -> Core controller: Torque,Power and Combined Torque/Power/4(n), Sum/2
  "Tr "/1 -> Core controller: Torque,Power and Combined Torque/Power/8(Tr)
  Core controller: Torque,Power and Combined Torque/Power/2(Qcp) -> Qcp/1
  Core controller: Torque,Power and Combined Torque/Power/1(Qcq) -> Qcq/1
  [eps_c] -> Core controller: Torque,Power and Combined Torque/Power/11(eps_c)
  [Ktr] -> Core controller: Torque,Power and Combined Torque/Power/12(K_t0r)
  [Kqr] -> Core controller: Torque,Power and Combined Torque/Power/13(K_q0r)

== system ctrl_T/Thruster control /Thruster 6/Thruster control/Core controller ==
  note: Core controller: Shaft speed
  n_r : Inport
  "Tr " : Inport  Port=2
  "n " : Inport  Port=3
  Core controller: Torque,Power and Combined Torque/Power : MATLAB Function  TreatAsAtomicUnit=on
  Integrator : Integrator  ExternalReset=either  UpperSaturationLimit=Q_max  LowerSaturationLimit=-Q_max
  Ki : Gain  Gain=Kp/0.05
  Kp : Gain  Gain=Kp
  Sum : Sum  Inputs=+|-
  Sum1 : Sum  Inputs=|++
  reset : S-Function  Priority=1  FunctionName=NIVeriStandIO  Parameters=width dtype portnum stime stype btype  mask(NI VeriStand Inport){portnum=1, width=-1, stime=-1, dtype=auto, stype=auto, btype=1}
      mask prompts: portnum "Port number:"; width "Port dimensions (-1 for dynamically sized):"; stime "Sample time (-1 for inherited):"; dtype "Data type:"; stype "Signal type:"; btype "Block type:"
      mask help: Use this inport on any level of nested subsystems to allow NI VeriStand software to map signals to it.
      mask init:
      | NIVeriStandIO_init;
      settings: CopyFcn=NIVeriStand_MDL_functions('', 'IO_copy');  DeleteFcn=NIVeriStand_MDL_functions('', 'IO_delete');  MoveFcn=set_param(gcb, 'Mask', 'on');
      mask Callback portnum: NIVeriStand_MDL_functions('', 'IO_setportnum');
      mask TypeOptions dtype: auto | double | single | int8 | uint8 | int16 | uint16 | int32 | uint32 | boolean
      mask Callback dtype: NIVeriStand_MDL_functions('', 'IO_booleansignal');
      mask TypeOptions stype: auto | real | complex
      mask Display:
      | patch([-x x], [-y y], [.90980 .81960 .32156]);
      | plot([xrad -x x xrad], [yrad -y y yrad]);
      | fprintf('NI In%d', portnum);
  Q_cn : Outport
  Qcq : Outport  Port=2
  Qcp : Outport  Port=3
  Qcc : Outport  Port=4
  wires:
  n_r/1 -> Sum/1
  Ki/1 -> Integrator/1
  Kp/1 -> Sum1/1
  Integrator/1 -> Sum1/2
  Sum/1 -> Ki/1, Kp/1
  Sum1/1 -> Q_cn/1
  reset/1 -> Integrator/2
  [k_cc] -> Core controller: Torque,Power and Combined Torque/Power/1(k_cc)
  [p_cc] -> Core controller: Torque,Power and Combined Torque/Power/2(p_cc)
  [r_cc] -> Core controller: Torque,Power and Combined Torque/Power/3(r_cc)
  Core controller: Torque,Power and Combined Torque/Power/3(Qcc) -> Qcc/1
  [Kt] -> Core controller: Torque,Power and Combined Torque/Power/5(K_t0)
  [D] -> Core controller: Torque,Power and Combined Torque/Power/7(D)
  [Kq] -> Core controller: Torque,Power and Combined Torque/Power/6(K_q0)
  [Rho] -> Core controller: Torque,Power and Combined Torque/Power/10(rho)
  [eps] -> Core controller: Torque,Power and Combined Torque/Power/9(eps)
  "n "/1 -> Core controller: Torque,Power and Combined Torque/Power/4(n), Sum/2
  "Tr "/1 -> Core controller: Torque,Power and Combined Torque/Power/8(Tr)
  Core controller: Torque,Power and Combined Torque/Power/2(Qcp) -> Qcp/1
  Core controller: Torque,Power and Combined Torque/Power/1(Qcq) -> Qcq/1
  [eps_c] -> Core controller: Torque,Power and Combined Torque/Power/11(eps_c)
  [Ktr] -> Core controller: Torque,Power and Combined Torque/Power/12(K_t0r)
  [Kqr] -> Core controller: Torque,Power and Combined Torque/Power/13(K_q0r)

== matlab function ctrl_T/TAPM Controller w_observer/LQR/MATLAB Function2 ==
  data: u input; y output
function y = fcn(u)
%#codegen

if u(1) < 0
    tau_x = 0;
else 
    tau_x = u(1);
end

    

y = [tau_x u(2) u(3)];

== matlab function ctrl_T/TAPM Controller w_observer/SP Generator/Set-Point Limiter ==
  data: sp input; sp_new output; fzp input; rmax input
function sp_new = spLimiter(sp,fzp,rmax)

sptofzp = sp-fzp;
offset = norm(sptofzp);
direction = sptofzp/offset; 
difference = sptofzp - rmax*direction; 
limit = (offset/rmax)^5;


    if (limit > 1) 
        limit = 1; 
    end 

sp_new = fzp+sptofzp-(limit*difference);
end

== matlab function ctrl_T/TAPM Controller w_observer/LQR/MATLAB Function3 ==
  data: r input; tau output; x_hat input; bias input
function tau = fcn(r,x_hat,bias)

K =[    6.4399         0         0   41.7347         0         0
         0    1.7636    -0.0044         0   24.5829    0.1054
         0   0.0015    5.0912         0   0.0663    28.4457];

P =[    6.4399         0         0
         0    1.7636  -0.0044
         0   0.0015    5.0912];

psi = x_hat(3);     

R  = [cos(psi) -sin(psi) 0;
        sin(psi) cos(psi) 0
        0           0      1];     

tau = P*r-K*x_hat-R\bias;

end

== matlab function ctrl_T/Thrust allocation1/For Each Subsystem/MATLAB Function ==
  data: angle input; y output
function y = rad2pipi(angle)
% RAD2PIPI Converts an angle in rad to the interval (-pi pi]
%          Should be applied to all heading errors in a feedback control system
%          in order to avoid discontinuities.
%
% Author:     Roger Skjetne
% Date:       2003-09-05
% Revisions:  2004-09-02 Thor I. Fossen - replaced input argument x with angle
%             2005-01-05 Thor I. Fossen - ouput argument is set to y and not angle
%             2005-04-13 Roger Skjetne  - changed the function s in order
%                                         to account for correct mapping to
%                                         (-pi pi].
%
% ________________________________________________________________
%
% MSS GNC is a Matlab toolbox for guidance, navigation and control.
% The toolbox is part of the Marine Systems Simulator (MSS).
%
% Copyright (C) 2008 Thor I. Fossen and Tristan Perez
% 
% This program is free software: you can redistribute it and/or modify
% it under the terms of the GNU General Public License as published by
% the Free Software Foundation, either version 3 of the License, or
% (at your option) any later version.
% 
% This program is distributed in the hope that it will be useful, but
% WITHOUT ANY WARRANTY; without even the implied warranty of
% MERCHANTABILITY or FITNESS FOR A PARTICULAR PURPOSE.  See the 
% GNU General Public License for more details.
% 
% You should have received a copy of the GNU General Public License
% along with this program.  If not, see <http://www.gnu.org/licenses/>.
% 
% E-mail: contact@marinecontrol.org
% URL:    <http://www.marinecontrol.org>


% convert angle in rad to the interval <-pi pi> 
r = rem(angle+sign(angle)*pi,2*pi);
s = sign(sign(angle) + 2*(sign(abs(rem(angle+pi,2*pi)/(2*pi)))-1));
% s = sign(angle);

y = r - s*pi;

== matlab function ctrl_T/TAPM Controller w_observer/surgeswaydampingrestoring ==
  data: r input; tau output; x_hat input; bias input
function tau = fcn(r,x_hat,bias)

K =[    0.5091         0         0   11.5609         0         0
         0    0.5091    0.0012         0   12.6308    0.0677
         0   -0.0012    0.5091         0   0.0157    8.7054];

P =[    0.5091         0         0
         0    0.5091  0.0012
         0   -0.0012    0.5091];

psi = x_hat(3);     

R  = [cos(psi) -sin(psi) 0;
        sin(psi) cos(psi) 0
        0           0      1];     

tau = P*r-K*x_hat;

end

== matlab function ctrl_T/Thrust allocation1/For Each Subsystem/MATLAB Function1 ==
  data: desired input; psi_D output; actual input
function psi_D   = fcn(desired,actual)
%#codegen
psi_D = desired-actual;
if abs(psi_D) >= 360
    psi_D = rem(psi_D,360);
end

if abs(psi_D) >= 180
    psi_D = psi_D - sign(psi_D)*360;
end

% if desired < 0 %&& abs(desired+actual) > 180
%     y = actual+360;
% else
%     y = abs(actual);
% end

%if desired-actual > 180
%    u = desired - 360;
%elseif desired-actual <= -180
%    u=actual + 360 ;
%else
%    u=desired;        
%end

end

%rotation = change-actual;% - actual; % If positive with clock, Negative against clock
%if rotation >= 180 || rotation <= -180
% u = desired;
%else 
%     u = actual;
%end

%change = abs(actual);

% if actual-desired > 180 && desired > 0 && rotation > 0
%     u = -180;
% elseif  actual-desired > 180 && desired > 0 && rotation < 0
%     u = 180;
% else 
%     u = actual;
% end

% if change > abs(desired-actual)
%     u = -actual;
% else
%     u = actual;
% end
% if desired >= 0.98*actual || desired <= -0.98*actual 
%     u = desired;
% else 
%     u = actual; 
% end
% paths = [abs(actual-desired),abs(-1*actual-desired)];
% fastest = min(paths);
% if paths(1) > paths(2)
%     fastest = paths(2);
% elseif paths(1) < paths(2)
%     fastest = paths(1);
% end
% % if desired > 0 && actual < 0 || desired < 0 && actual < 0
% % u = fastest;
% % elseif desired > 0 && actual > 0 || desired < 0 && actual < 0
% %     u = fastest;
% if desired-actual > 180 || desired-actual < -180
%     u = -actual;
% else 
%     u = actual;
% end

== matlab function ctrl_T/Thrust allocation1/MATLAB Function ==
  data: u input; sys output; ThrusterPosX input; ThrusterPosY input; C input
function sys = fcn(u,ThrusterPosX,ThrusterPosY,C)
% Complete system goes here!
Alpha1 = zeros(1,6);
% ThrusterPosX = [Thruster.T1(1) Thruster.T2(1) Thruster.T3(1) Thruster.T4(1) Thruster.T5(1) Thruster.T6(1)];%[x(1),x(2),x(3),x(4),x(5),x(6)]';
% ThrusterPosY = [Thruster.T1(2) Thruster.T2(2) Thruster.T3(2) Thruster.T4(2) Thruster.T5(2) Thruster.T6(2)];%[x(7),x(8),x(9),x(10),x(11),x(12)]';
% Parameters thrusters
tc =  [u(1),u(2),u(3)]'; 
alpha = [u(4),u(5),u(6),u(7),u(8),u(9)]';
%alpha0 = [x(1),x(2),x(3),x(4),x(5),x(6)]';

% Constraints for Thruster-Thruster interaction. Can be seen in "Initfile"
% how they are found
C1 = C(1,:);
C2 = C(2,:);
C3 = C(3,:);
C4 = C(4,:);
C5 = C(5,:);
C6 = C(6,:);


K = ones(1,6);
% 
% % Ok 12.05/16
% if (alpha(1) < C1(1)-0.1  && alpha(1) > C1(2)+0.1) || (alpha(1) > C1(3)+0.1 && alpha(1) < C1(4)-0.1)
%     K(1) = 0;
% else 
%     K(1) = K(1);
% end
% % OK 12.05/16
% if (alpha(2) < C2(1)-0.1  && alpha(2) > C2(2)+0.1) || (alpha(2) < C2(3)-0.1 && alpha(2) > C2(4)+0.1)
%     K(2) = 0;
% else 
%     K(2) = K(2);
% end
% % OK 12.05/16
% if (alpha(3) > C3(1)+0.1  && alpha(3) < C3(2)-0.1) || (alpha(3) > C3(3)+0.1 && alpha(3) < C3(4)-0.1)
%     K(3) = 0;
% else 
%     K(3) = K(3);
% end
% % OK 12.05/16
% if (alpha(4) > C4(1)+0.1  && alpha(4) < C4(2)-0.1) || (alpha(4) < C4(3)- 0.1 && alpha(4) > C4(4)+0.1)
%     K(4) = 0;
% else 
%     K(4) = K(4);
% end
% % OK 12.05/16
% if (alpha(5) > C5(1)+0.1  && alpha(5) < C5(2)-0.1) || (alpha(5) > C5(3)+0.1 && alpha(5) < C5(4)-0.1)
%     K(5) = 0;
% else 
%     K(5) = K(5);
% end
% % OK 12.05/16
% if (alpha(6) < C6(1)-0.1  && alpha(6) > C6(2)+0.1) || (alpha(6) < C6(3)-0.1 && alpha(6) > C6(4)+0.1)
%     K(6) = 0;
% else 
%     K(6) = K(6);
% end
% 
% K = [K(1) K(2) K(3) K(4) K(5) K(6)];

n_t = length(ThrusterPosX); % number of thrusters
T_surge = zeros(n_t,1); % Shells for faster computing
T_sway = zeros(n_t,1);  % Shells for faster computing
T_yaw = zeros(n_t,1);   % Shells for faster computing

for i = 1:1:n_t
  T_surge(i) = cosd(alpha(i));     %Thrust in x-direction for cartesian
  T_sway(i) = sind(alpha(i));      %Thrust in y-direction for cartesian
  T_yaw(i) = (sind(alpha(i))*ThrusterPosX(i) - cosd(alpha(i))*ThrusterPosY(i));
end


B = [T_surge,T_sway,T_yaw]';
B = B*diag(K); 
[U_singular,S_singular,V_singular] = svd(B,'econ');
S_singular_cross = 1./S_singular;
S_singular_cross(~isfinite(S_singular_cross))=0;
 if (S_singular_cross(3,3)>2*S_singular_cross(2,2)) 
     S_singular_cross(3,3)=0;
 end

T_optimized = V_singular*S_singular_cross*U_singular';
T_d = T_optimized*tc;          % Optimized Thrust

 


Te = [1 0 1 0 1 0 1 0 1 0 1 0;
      0 1 0 1 0 1 0 1 0 1 0 1;
      ThrusterPosY(1) ThrusterPosX(1) ThrusterPosY(2) ThrusterPosX(2) ThrusterPosY(3) ThrusterPosX(3) ...
      ThrusterPosY(4) ThrusterPosX(4) ThrusterPosY(5) ThrusterPosX(5) ThrusterPosY(6) ThrusterPosX(6)];

[U_singular,S_singular,V_singular] = svd(Te,'econ');
S_singular_cross = 1./S_singular;
S_singular_cross(~isfinite(S_singular_cross))=0;
 if (S_singular_cross(3,3)>2*S_singular_cross(2,2)) 
     S_singular_cross(3,3)=0;
 end
T0 = V_singular*S_singular_cross*U_singular'*tc;

alpha1 = [atan2d(T0(2),T0(1)) atan2d(T0(4),T0(3)) atan2d(T0(6),T0(5)) atan2d(T0(8),T0(7)) atan2d(T0(10),T0(9)) atan2d(T0(12),T0(11))];
%alpha1 = [ 180 -90 90 0 25 -25];
% for i=1:1:n_t
%   if alpha1(i) > 180
%       alpha1(i) = alpha1(i) - 360;
%   elseif alpha1(i) < -180
%       alpha1(i) = alpha1(i) + 360;
%   else
%       alpha1(i) = alpha(i);
%   end
% end

%alpha1 = [180 -90 90 atan2d(T0(8),T0(7)) 0 0];

%% Constraints
% % Thruster 1 OK 13.05/16
% % %C1 = [49.7 29.4 -151 -130 ];
% 
% if (alpha1(1) < C1(1)  && alpha1(1) > C1(2)) %&& T_d(1) > 0) || (alpha1(1) < C1(1)  && alpha1(1) > C1(2) && T_d(1) < 0)
%     c1 = [C1(1) C1(2)];
%     [C_1,alpha_new1] = min(abs(c1-alpha1(1)));
%     Alpha1(1) = c1(alpha_new1);
% elseif (alpha1(1) > C1(3) && alpha1(1) < C1(4) && T_d(1) > 0) || (alpha1(1) > C1(3) && alpha1(1) < C1(4) && T_d(1) < 0)
%     c1 = [C1(3) C1(4)];
%     [C_1,alpha_new1] = min(abs(c1-alpha1(1)));
%     Alpha1(1) = c1(alpha_new1);
% else 
%     Alpha1(1) = alpha1(1);
% end
% if alpha(1) < C1(1)-0.1  && alpha(1) > C1(2)+0.1 || alpha(1) > C1(3)+0.1 && alpha(1) < C1(4)-0.1
%     T_d(1) = 0;
% else 
%     T_d(1) = T_d(1);
% end
%  
% %% Thruster 2 OK 13.05/16
% %C2 = [99.85 80.15 50 29];
% if (alpha1(2) < C2(1)  && alpha1(2) > C2(2) && T_d(2) > 0) || (alpha1(2) < C2(1)  && alpha1(2) > C2(2) && T_d(2) < 0) 
%     c2 = [C2(1) C2(2)];
%     [C_2,alpha_new2] = min(abs(c2-alpha1(2)));
%     Alpha1(2) = c2(alpha_new2);
% elseif (alpha1(2) < C2(3) && alpha1(2) > C2(4) && T_d(2) > 0) || (alpha1(2) < C2(3) && alpha1(2) > C2(4) && T_d(2) < 0)
%     c2 = [C2(3) C2(4)];
%     [C_2,alpha_new2] = min(abs(c2-alpha1(2)));
%     Alpha1(2) = c2(alpha_new2);
% else 
%     Alpha1(2) = alpha1(2);
% end
% if (alpha(2) < C2(1)-0.1  && alpha(2) > C2(2)+0.1) || (alpha(2) < C2(3)-0.1 && alpha(2) > C2(4)+0.1)
%     T_d(2) = 0;
% else 
%     T_d(2) = T_d(2);
% end
% 
% %% Thruster 3 OK 13.05/16
% % C3 = [-99.85 -80.15 -50 -29]; 
% 
% if (alpha1(3) > C3(1)  && alpha1(3) < C3(2) && T_d(3) > 0) || (alpha1(3) > C3(1)  && alpha1(3) < C3(2) && T_d(3) < 0)
%     c3 = [C3(1) C3(2)];
%     [C_3,alpha_new3] = min(abs(c3-alpha1(3)));
%     Alpha1(3) = c3(alpha_new3);
% elseif (alpha1(3) > C3(3) && alpha1(3) < C3(4) && T_d(3) > 0) || (alpha1(3) > C3(3) && alpha1(3) < C3(4) && T_d(3) < 0) 
%     c3 = [C3(3) C3(4)];
%     [C_3,alpha_new3] = min(abs(c3-alpha1(3)));
%     Alpha1(3) = c3(alpha_new3);
% else 
%     Alpha1(3) = alpha1(3);
% end
% if (alpha(3) > C3(1) + 0.1  && alpha(3) < C3(2) - 0.1) || (alpha(3) > C3(3) + 0.1 && alpha(3) < C3(4) - 0.1)
%     T_d(3) = 0;
% else 
%     T_d(3) = T_d(3);
% end
% 
% %% Thruster 4 OK 13.05/16
% %C4 = [-52.8 -34.2 52.8 34.2]; 
% if (alpha1(4) > C4(1)  && alpha1(4) < C4(2) && T_d(4) > 0) || (alpha1(4) > C4(1)  && alpha1(4) < C4(2) && T_d(4) < 0)
%     c4 = [C4(1) C4(2)];
%     [C_4,alpha_new4] = min(abs(c4-alpha1(4)));
%     Alpha1(4) = c4(alpha_new4);
% elseif (alpha1(4) < C4(3) && alpha1(4) > C4(4) && T_d(4) > 0) || (alpha1(4) < C4(3) && alpha1(4) > C4(4) && T_d(4) < 0) 
%     c4 = [C4(3) C4(4)];
%     [C_4,alpha_new4] = min(abs(c4-alpha1(4)));
%     Alpha1(4) = c4(alpha_new4);
% else 
%     Alpha1(4) = alpha1(4);
% end
% if (alpha(4) > C4(1)+0.1  && alpha(4) < C4(2)-0.1) || (alpha(4) < C4(3)-0.1 && alpha(4) > C4(4)+0.1)
%     T_d(4) = 0;
% else 
%     T_d(4) = T_d(4);
% end
% 
% %% Thruster 5 OK 13.05/16
% %C5 = [-98.25 -81.75 -145.8 -127.2];
% if (alpha1(5) > C5(1)  && alpha1(5) < C5(2) && T_d(5) > 0) || (alpha1(5) > C5(1)  && alpha1(5) < C5(2) && T_d(5) < 0)
%     c5 = [C5(1) C5(2)];
%     [C_5,alpha_new5] = min(abs(c5-alpha1(5)));
%     Alpha1(5) = c5(alpha_new5);
% elseif (alpha1(5) > C5(3) && alpha1(5) < C5(4) && T_d(5) > 0)  || (alpha1(5) > C5(3) && alpha1(5) < C5(4) && T_d(5) < 0)
%     c5 = [C5(3) C5(4)];
%     [C_5,alpha_new5] = min(abs(c5-alpha1(5)));
%     Alpha1(5) = c5(alpha_new5);
% else 
%     Alpha1(5) = alpha1(5);
% end
% if (alpha(5) > C5(1)+0.1  && alpha(5) < C5(2)-0.1) || (alpha(5) > C5(3)+0.1 && alpha(5) < C5(4)-0.1)
%     T_d(5) = 0;
% else 
%     T_d(5) = T_d(5);
% end
% 
% %% Thruster 6 OK 13.05/16
% %C6 = [98.75 81.75 145.8 127.2];
% if (alpha1(6) < C6(1)  && alpha1(6) > C6(2) && T_d(6) > 0) || (alpha1(6) < C6(1)  && alpha1(6) > C6(2) && T_d(6) < 0)
%     c6 = [C6(1) C6(2)];
%     [C_6,alpha_new6] = min(abs(c6-alpha1(6)));
%     Alpha1(6) = c6(alpha_new6);
% elseif (alpha1(6) < C6(3) && alpha1(6) > C6(4) && T_d(6) > 0) || (alpha1(6) < C6(3) && alpha1(6) > C6(4) && T_d(6) < 0)
%     c6 = [C6(3) C6(4)];
%     [C_6,alpha_new6] = min(abs(c6-alpha1(6)));
%     Alpha1(6) = c6(alpha_new6);
% else 
%     Alpha1(6) = alpha1(6);
% end
% if (alpha(6) < C6(1)-0.1  && alpha(6) > C6(2)+0.1) || (alpha(6) < C6(3)-0.1 && alpha(6) > C6(4)+0.1)
%     T_d(6) = 0;
% else 
%     T_d(6) = T_d(6);
% end
% 
% % Thruster 2&3 
% if Alpha1(2) == C2(2)
%     Alpha1(3) = alpha1(2) - (C2(2) - alpha1(2));
% elseif Alpha1(2) == C2(1)
%     Alpha1(3) = alpha1(2) - (C2(1) - alpha1(2));
% elseif Alpha1(2) == C2(3)
%     Alpha1(3) = alpha1(2) - (C2(3) - alpha1(2));
% elseif Alpha1(2) == C2(4)
%     Alpha1(3) = alpha1(2) - (C2(4) - alpha1(2));
%     
% elseif Alpha1(3) == C3(2)
%     Alpha1(2) = alpha1(3) - (C3(2) - alpha1(3));
% elseif Alpha1(3) == C3(1)
%     Alpha1(2) = alpha1(3) - (C3(1) - alpha1(3));
% elseif Alpha1(3) == C3(3)
%     Alpha1(2) = alpha1(3) - (C3(3) - alpha1(3));
% elseif Alpha1(3) == C3(4)
%     Alpha1(2) = alpha1(3) - (C3(4) - alpha1(3));
% end
% 
% % Thruster 5&6
% if Alpha1(5) == C5(2)
%     Alpha1(6) = alpha1(5) - (C5(2) - alpha1(5));
% elseif Alpha1(5) == C5(1)
%     Alpha1(6) = alpha1(5) - (C5(1) - alpha1(5));
% elseif Alpha1(5) == C5(3)
%     Alpha1(6) = alpha1(5) - (C5(3) - alpha1(5));
% elseif Alpha1(5) == C5(4)
%     Alpha1(6) = alpha1(5) - (C5(4) - alpha1(5));
%     
% elseif Alpha1(6) == C6(2)
%     Alpha1(5) = alpha1(6) - (C6(2) - alpha1(6));
% elseif Alpha1(6) == C6(1)
%     Alpha1(5) = alpha1(6) - (C6(1) - alpha1(6));
% elseif Alpha1(6) == C6(3)
%     Alpha1(5) = alpha1(6) - (C6(3) - alpha1(6));
% elseif Alpha1(6) == C6(4)
%     Alpha1(5) = alpha1(6) - (C6(4) - alpha1(6));
% end
% % Thruster 4 & 1
% if     Alpha1(4) == C4(2)
%     Alpha1(1) = alpha1(4) - (C4(2) - alpha1(4));
% elseif Alpha1(4) == C4(1)
%     Alpha1(1) = alpha1(4) - (C4(1) - alpha1(4));
% elseif Alpha1(4) == C4(3)
%     Alpha1(1) = alpha1(4) - (C4(3) - alpha1(4));
% elseif Alpha1(4) == C4(4)
%     Alpha1(1) = alpha1(4) - (C4(4) - alpha1(4));
% end
% 
% if     Alpha1(1) == C1(2)
%     Alpha1(4) = alpha1(1) - (C1(2) - alpha1(1));
% elseif Alpha1(1) == C1(1)
%     Alpha1(4) = alpha1(1) - (C1(1) - alpha1(1));
% elseif Alpha1(1) == C1(3)
%     Alpha1(4) = alpha1(1) - (C1(3) - alpha1(1));
% elseif Alpha1(1) == C1(4)
%     Alpha1(4) = alpha1(1) - (C1(4) - alpha1(1));
% end
% 
% Alpha1 = [Alpha1(1) Alpha1(2) Alpha1(3) Alpha1(4) Alpha1(5) Alpha1(6)]';    
% Desired_thrust = [T_d(1) T_d(2) T_d(3) T_d(4) T_d(5) T_d(6)]';
% alpha_desired = Alpha1;

% T_d = -Desired_thrust;
%% Update outputs
sys = [alpha1,T_d']';
